simulink model "izaje_carro"  (R2019a)
settings: Solver=VariableStepAuto  StartTime=0.0  StopTime=10.0  RelTol=1e-3
values from neighbouring files (symbols this model uses):
  b_h_eq = 2 * ( b_hd + i_h^2*b_hm ) / (r_hd^2)    (= 31004.4444444)    [parametros.m]
  b_hb = 1.0e8    (= 100000000)    [parametros.m]
  b_hEb = 2.2e9    (= 2200000000)    [parametros.m]
  b_wu = 150    [parametros.m]
  i_h = 22.0    (= 22)    [parametros.m]
  k_wu = 2.36e8    (= 236000000)    [parametros.m]
  l_h0 = Y_t0 - y_h0    [parametros.m]
  m_h_eq = 2 * ( J_hd_hEb + i_h^2*J_hm_hb ) / (r_hd^2)    (= 65137.7777778)    [parametros.m]
  r_hd = 0.75    [parametros.m]
  T_hb_max = 5.0e4    (= 50000)    [parametros.m]
  T_hEb_max = 1.1e6    (= 1100000)    [parametros.m]
settings Model: Creator=Adrián  LastModifiedBy=Facundo

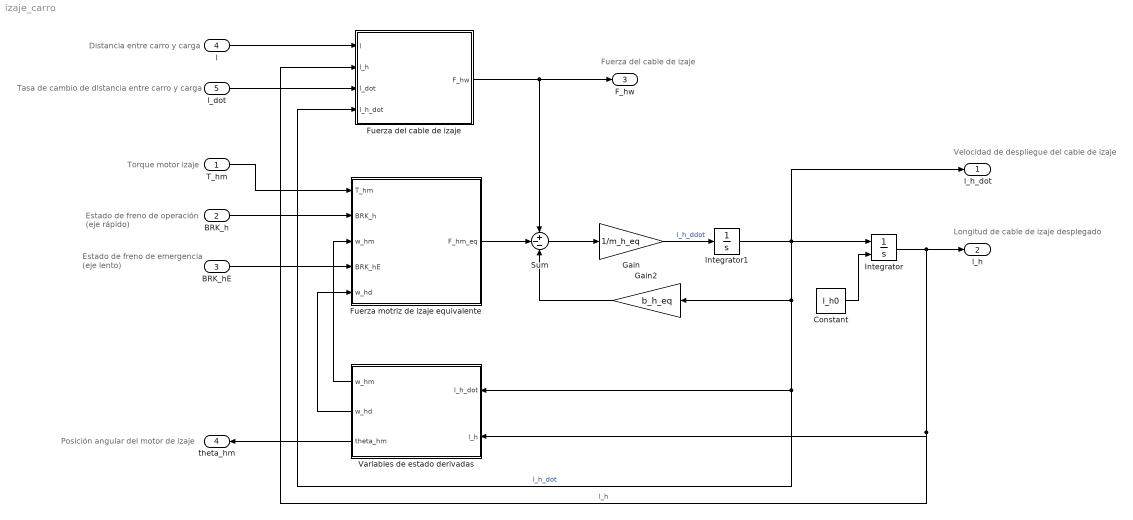
== system izaje_carro ==
  note: Estado de freno de emergencia
      | (eje lento)
  note: Fuerza del cable de izaje
  note: Longitud de cable de izaje desplegado
  note: Velocidad de despliegue del cable de izaje
  note: Estado de freno de operación
      | (eje rápido)
  note: Distancia entre carro y carga
  note: Posición angular del motor de izaje
  note: Tasa de cambio de distancia entre carro y carga
  note: Torque motor izaje
  T_hm : Inport
  BRK_h : Inport  Port=2
  BRK_hE : Inport  Port=3
  l : Inport  Port=4
  l_dot : Inport  Port=5
  Constant : Constant  Value=l_h0
  Fuerza del cable de izaje : Subsystem
  Fuerza motriz de izaje equivalente : Subsystem
  Gain : Gain  Gain=1/m_h_eq
  Gain2 : Gain  Gain=b_h_eq
  Integrator : Integrator  InitialConditionSource=external
  Integrator1 : Integrator
  Sum : Sum  Inputs=+--
  Variables de estado derivadas : Subsystem
  l_h_dot : Outport
  l_h : Outport  Port=2
  F_hw : Outport  Port=3
  theta_hm : Outport  Port=4
  wires:
  Variables de estado derivadas/3(theta_hm) -> theta_hm/1
  Gain/1 -> Integrator1/1  "l_h_ddot"
  Constant/1 -> Integrator/2
  Variables de estado derivadas/2(w_hd) -> Fuerza motriz de izaje equivalente/5(w_hd)
  BRK_h/1 -> Fuerza motriz de izaje equivalente/2(BRK_h)
  BRK_hE/1 -> Fuerza motriz de izaje equivalente/4(BRK_hE)
  Sum/1 -> Gain/1
  Variables de estado derivadas/1(w_hm) -> Fuerza motriz de izaje equivalente/3(w_hm)
  Gain2/1 -> Sum/3
  Integrator1/1 -> l_h_dot/1, Fuerza del cable de izaje/4(l_h_dot), Variables de estado derivadas/1(l_h_dot), Gain2/1, Integrator/1  "l_h_dot"
  Fuerza del cable de izaje/1(F_hw) -> F_hw/1, Sum/1
  Fuerza motriz de izaje equivalente/1(F_hm_eq) -> Sum/2
  l/1 -> Fuerza del cable de izaje/1(l)
  T_hm/1 -> Fuerza motriz de izaje equivalente/1(T_hm)
  Integrator/1 -> l_h/1, Variables de estado derivadas/2(l_h), Fuerza del cable de izaje/2(l_h)  "l_h"
  l_dot/1 -> Fuerza del cable de izaje/3(l_dot)

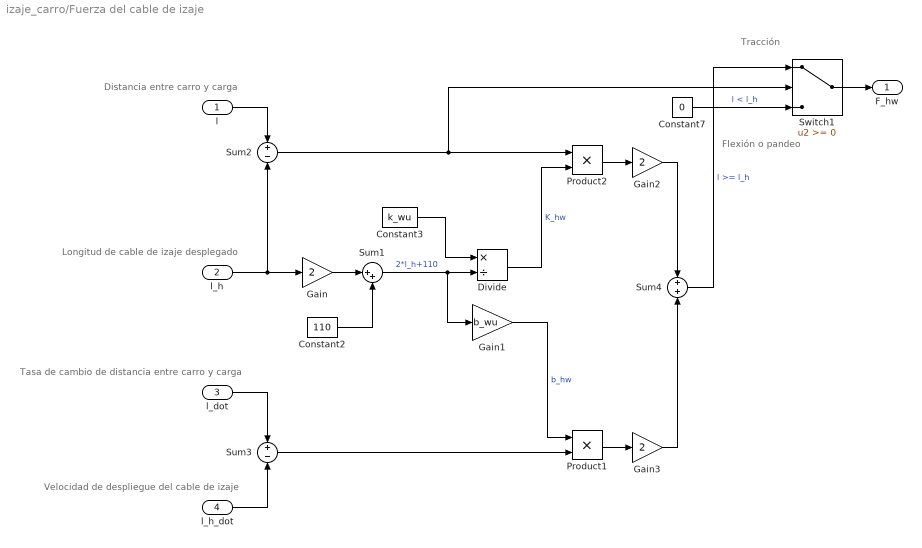
== system izaje_carro/Fuerza del cable de izaje ==
  note: Flexión o pandeo
  note: Tracción
  note: Distancia entre carro y carga
  note: Tasa de cambio de distancia entre carro y carga
  note: Longitud de cable de izaje desplegado
  note: Velocidad de despliegue del cable de izaje
  l : Inport
  l_h : Inport  Port=2
  l_dot : Inport  Port=3
  l_h_dot : Inport  Port=4
  Constant2 : Constant  Value=110
  Constant3 : Constant  Value=k_wu
  Constant7 : Constant  Value=0
  Divide : Product  Inputs=*/
  Gain : Gain  Gain=2
  Gain1 : Gain  Gain=b_wu
  Gain2 : Gain  Gain=2
  Gain3 : Gain  Gain=2
  Product1 : Product
  Product2 : Product
  Sum1 : Sum  Inputs=|++
  Sum2 : Sum  Inputs=+-
  Sum3 : Sum  Inputs=+-
  Sum4 : Sum
  Switch1 : Switch
  F_hw : Outport
  wires:
  l_dot/1 -> Sum3/1
  Constant2/1 -> Sum1/2
  Sum1/1 -> Gain1/1, Divide/2  "2*l_h+110"
  l/1 -> Sum2/1
  Product1/1 -> Gain3/1
  Sum3/1 -> Product1/2
  l_h_dot/1 -> Sum3/2
  l_h/1 -> Gain/1, Sum2/2
  Divide/1 -> Product2/2  "K_hw"
  Sum2/1 -> Switch1/2, Product2/1
  Constant3/1 -> Divide/1
  Gain1/1 -> Product1/1  "b_hw"
  Product2/1 -> Gain2/1
  Switch1/1 -> F_hw/1
  Sum4/1 -> Switch1/1  "l >= l_h"
  Constant7/1 -> Switch1/3  "l < l_h"
  Gain/1 -> Sum1/1
  Gain2/1 -> Sum4/1
  Gain3/1 -> Sum4/2

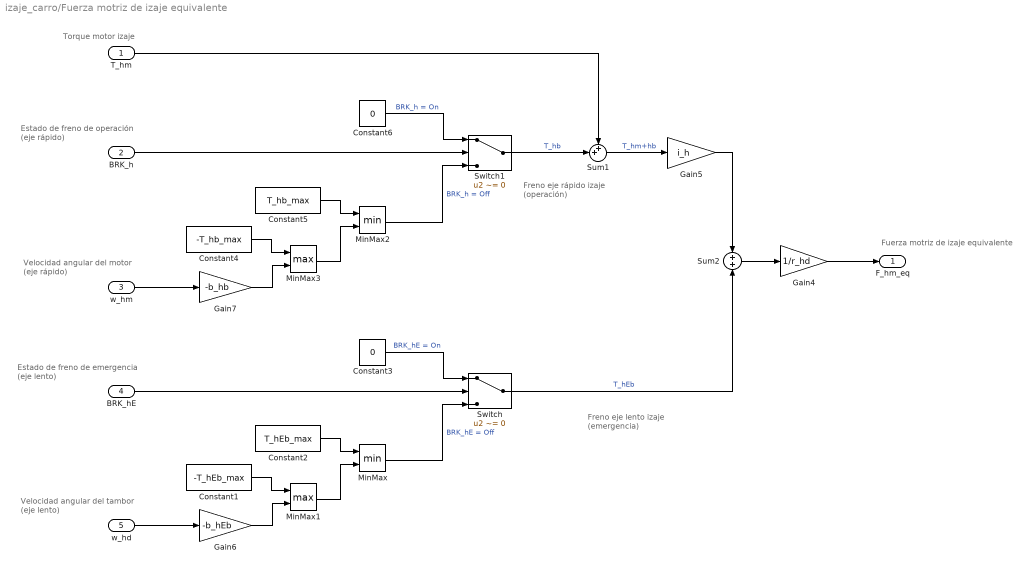
== system izaje_carro/Fuerza motriz de izaje equivalente ==
  note: Fuerza motriz de izaje equivalente
  note: Torque motor izaje
  note: Freno eje lento izaje
      | (emergencia)
  note: Freno eje rápido izaje
      | (operación)
  note: Estado de freno de operación
      | (eje rápido)
  note: Estado de freno de emergencia
      | (eje lento)
  note: Velocidad angular del tambor
      | (eje lento)
  note: Velocidad angular del motor
      | (eje rápido)
  T_hm : Inport
  BRK_h : Inport  Port=2  OutDataTypeStr=boolean
  w_hm : Inport  Port=3
  BRK_hE : Inport  Port=4  OutDataTypeStr=boolean
  w_hd : Inport  Port=5
  Constant1 : Constant  Value=-T_hEb_max
  Constant2 : Constant  Value=T_hEb_max
  Constant3 : Constant  Value=0
  Constant4 : Constant  Value=-T_hb_max
  Constant5 : Constant  Value=T_hb_max
  Constant6 : Constant  Value=0
  Gain4 : Gain  Gain=1/r_hd
  Gain5 : Gain  Gain=i_h
  Gain6 : Gain  Gain=-b_hEb
  Gain7 : Gain  Gain=-b_hb
  MinMax : MinMax  Inputs=2
  MinMax1 : MinMax  Function=max  Inputs=2
  MinMax2 : MinMax  Inputs=2
  MinMax3 : MinMax  Function=max  Inputs=2
  Sum1 : Sum  Inputs=++|
  Sum2 : Sum  Inputs=2
  Switch : Switch  Criteria=u2 ~= 0
  Switch1 : Switch  Criteria=u2 ~= 0
  F_hm_eq : Outport
  wires:
  MinMax3/1 -> MinMax2/2
  MinMax1/1 -> MinMax/2
  Constant1/1 -> MinMax1/1
  MinMax2/1 -> Switch1/3  "BRK_h = Off"
  Gain5/1 -> Sum2/1
  Constant4/1 -> MinMax3/1
  T_hm/1 -> Sum1/1
  w_hm/1 -> Gain7/1
  Constant5/1 -> MinMax2/1
  w_hd/1 -> Gain6/1
  Gain7/1 -> MinMax3/2
  BRK_h/1 -> Switch1/2
  Constant6/1 -> Switch1/1  "BRK_h = On"
  MinMax/1 -> Switch/3  "BRK_hE = Off"
  Sum1/1 -> Gain5/1  "T_hm+hb"
  Switch1/1 -> Sum1/2  "T_hb"
  Constant3/1 -> Switch/1  "BRK_hE = On"
  BRK_hE/1 -> Switch/2
  Constant2/1 -> MinMax/1
  Gain6/1 -> MinMax1/2
  Gain4/1 -> F_hm_eq/1
  Sum2/1 -> Gain4/1
  Switch/1 -> Sum2/2  "T_hEb"

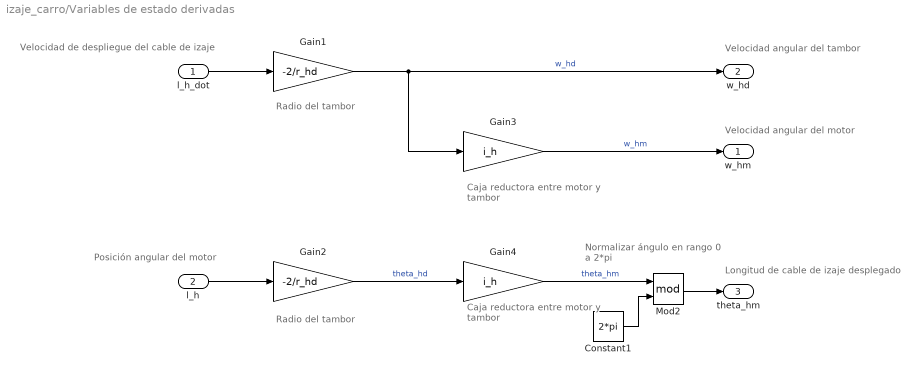
== system izaje_carro/Variables de estado derivadas ==
  note: Velocidad angular del tambor
  note: Caja reductora
      | entre motor y tambor
  note: Velocidad angular del motor
  note: Velocidad de despliegue del cable de izaje
  note: Longitud de cable de izaje desplegado
  note: Posición angular del motor
  note: Caja reductora
      | entre motor y tambor
  note: Radio del tambor
  note: Radio del tambor
  note: Normalizar ángulo en
      | rango 0 a 2*pi
  l_h_dot : Inport
  l_h : Inport  Port=2
  Constant1 : Constant  Value=2*pi
  Gain1 : Gain  Gain=-2/r_hd
  Gain2 : Gain  Gain=-2/r_hd
  Gain3 : Gain  Gain=i_h
  Gain4 : Gain  Gain=i_h
  Mod2 : Math  Operator=mod  SaturateOnIntegerOverflow=on
  w_hm : Outport
  w_hd : Outport  Port=2
  theta_hm : Outport  Port=3
  wires:
  Gain1/1 -> w_hd/1, Gain3/1  "w_hd"
  l_h_dot/1 -> Gain1/1
  Gain3/1 -> w_hm/1  "w_hm"
  Gain2/1 -> Gain4/1  "theta_hd"
  l_h/1 -> Gain2/1
  Gain4/1 -> Mod2/1  "theta_hm"
  Constant1/1 -> Mod2/2
  Mod2/1 -> theta_hm/1
